simulink model "svpwm_inv_Motor_new_sent_split4"  (R2023a)
settings: Solver=daessc  StartTime=0.0  StopTime=0.62  MaxStep=2.5e-7  RelTol=1e-3
undefined symbols (not defined in the file): DiscIntNeverNeededParam
libraries: nesl_utility x37, fl_lib x34, ee_lib x21, spsMeanLib x7, simulink x6, mcbcontrolslib x4, slpidlib x4, sdl_lib x2, simulink_extras x1
(part 2 of 2)

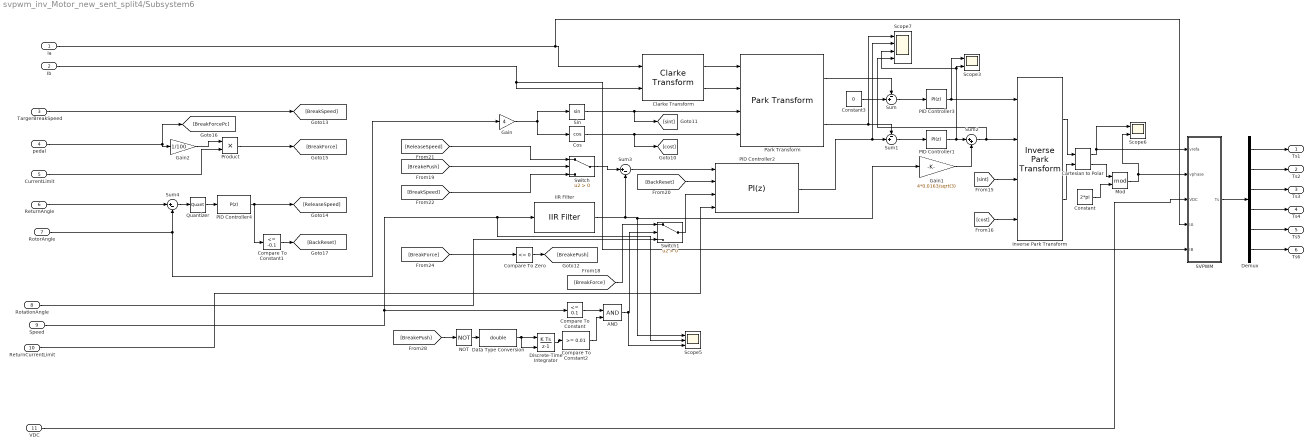
== system svpwm_inv_Motor_new_sent_split4/Subsystem6 ==
  Ia : Inport
  Ib : Inport  Port=2
  TargerBreakSpeed : Inport  Port=3
  pedal : Inport  Port=4
  CurrentLimit : Inport  Port=5
  ReturnAngle : Inport  Port=6
  RotorAngle : Inport  Port=7
  RotationAngle : Inport  Port=8
  Speed : Inport  Port=9
  ReturnCurrentLimit : Inport  Port=10
  VDC : Inport  Port=11
  AND : Logic  IconShape=distinctive  AllPortsSameDT=off  OutDataTypeStr=boolean
  Cartesian to Polar : simulink_extras/Transformations/Cartesian to Polar
  Clarke Transform : mcbcontrolslib/Clarke Transform  VariantControl=Variant2
      settings: LibrarySourceBlock=mcbhdllib/Controls/Math Transforms/Clarke Transform
  Compare To Constant : simulink/Logic and Bit Operations/Compare To Constant  relop=<=  const=0.1  OutDataTypeStr=boolean
  Compare To Constant1 : simulink/Logic and Bit Operations/Compare To Constant  relop=<=  const=-0.1  OutDataTypeStr=boolean
  Compare To Constant2 : simulink/Logic and Bit Operations/Compare To Constant  relop=>=  const=0.01  OutDataTypeStr=boolean
  Compare To Zero : simulink/Logic and Bit Operations/Compare To Zero  relop=<=  OutDataTypeStr=boolean
  Constant : Constant  Value=2*pi  SampleTime=-1
  Constant3 : Constant  Value=0  SampleTime=-1
  Cos : Trigonometry  Operator=cos
  Data Type Conversion : DataTypeConversion  OutDataTypeStr=double  SaturateOnIntegerOverflow=off  RndMeth=Floor
  Demux : Demux  Outputs=6
  Discrete-Time Integrator : DiscreteIntegrator  ExternalReset=rising  SampleTime=-1  ICPrevOutput=DiscIntNeverNeededParam  ICPrevScaledInput=DiscIntNeverNeededParam
  Gain : Gain  Gain=4
  Gain1 : Gain  Gain=4*0.0163/sqrt(3)
  Gain2 : Gain  Gain=1/100
  IIR Filter : mcbcontrolslib/IIR Filter  VariantControl=Low Pass Filter  VariantSelect=Low-pass  Filter_constant=7e-1  advancedSettings=off  Ts=50e-6  cutOff_freq=7427.2307
      settings: LibrarySourceBlock=mcbhdllib/Signal Management/IIR Filter
  Inverse Park Transform : mcbcontrolslib/Inverse Park Transform  AxisAlignment=D-axis
      settings: LibrarySourceBlock=mcbhdllib/Controls/Math Transforms/Inverse Park Transform
  Mod : Math  Operator=mod
  NOT : Logic  Operator=NOT  IconShape=distinctive  AllPortsSameDT=off  OutDataTypeStr=boolean
  PID Controller1 : slpidlib/PID Controller  Controller=PI  Form=Parallel  TimeDomain=Discrete-time  UseExternalTs=off  SampleTime=-1  IntegratorMethod=Forward Euler  FilterMethod=Forward Euler  ControllerParametersSource=internal  P=1*0.15  I=599*0.15  UseKiTs=off  D=0  N=100  UseFilter=on  TunerSelectOption=Transfer Function Based (PID Tuner App)  InitialConditionSource=internal  InitialConditionForIntegrator=0  InitialConditionForFilter=0  DifferentiatorICPrevScaledInput=0  ExternalReset=none  TrackingMode=off  Kt=1  LimitOutput=on  SatLimitsSource=internal  UpperSaturationLimit=15  LowerSaturationLimit=-15  LinearizeAsGain=off  AntiWindupMode=clamping  Kb=1  LimitIntegrator=off  UpperIntegratorSaturationLimit=inf  LowerIntegratorSaturationLimit=-inf  POutMin=[]  POutMax=[]  IOutMin=[]  IOutMax=[]  DOutMin=[]  DOutMax=[]  NOutMin=[]  NOutMax=[]  SumOutMin=[]  SumOutMax=[]  SaturationOutMin=[]  SaturationOutMax=[]  PParamMin=[]  PParamMax=[]  IParamMin=[]  IParamMax=[]  DParamMin=[]  DParamMax=[]  NParamMin=[]  NParamMax=[]  KbParamMin=[]  KbParamMax=[]  KtParamMin=[]  KtParamMax=[]  KbOutMin=[]  KbOutMax=[]  KtOutMin=[]  KtOutMax=[]  IntegratorOutMin=[]  IntegratorOutMax=[]  FilterOutMin=[]  FilterOutMax=[]  SumI1OutMin=[]  SumI1OutMax=[]  SumI2OutMin=[]  SumI2OutMax=[]  SumI3OutMin=[]  SumI3OutMax=[]  SumI4OutMin=[]  SumI4OutMax=[]  SumDOutMin=[]  SumDOutMax=[]  DifferentiatorOutMin=[]  DifferentiatorOutMax=[]  FilterDiffOutCoefMin=[]  FilterDiffOutCoefMax=[]  ReciprocalOutMin=[]  ReciprocalOutMax=[]  SumDenOutMin=[]  SumDenOutMax=[]  SumNumOutMin=[]  SumNumOutMax=[]  DivideOutMin=[]  DivideOutMax=[]  UdiffTsProdOutMin=[]  UdiffTsProdOutMax=[]  NTsProdOutMin=[]  NTsProdOutMax=[]  UintegralTsProdOutMin=[]  UintegralTsProdOutMax=[]  UngainTsProdOutMin=[]  UngainTsProdOutMax=[]  ClampingZeroOutDataTypeStr=Inherit: Inherit via back propagation  ClampingZeroOutMin=[]  ClampingZeroOutMax=[]  FilterDenConstantOutDataTypeStr=Inherit: Inherit via back propagation  FilterDenConstantOutMin=[]  FilterDenConstantOutMax=[]  PCopyOutDataTypeStr=Inherit: Inherit via back propagation  PCopyOutMin=[]  PCopyOutMax=[]  NCopyOutDataTypeStr=Inherit: Inherit via back propagation  NCopyOutMin=[]  NCopyOutMax=[]  IntegratorContinuousStateAttributes=''  IntegratorStateMustResolveToSignalObject=off  IntegratorRTWStateStorageClass=Auto  FilterContinuousStateAttributes=''  FilterStateMustResolveToSignalObject=off  FilterRTWStateStorageClass=Auto  ParallelPVariant=InternalParameters  IdealPVariant=Disabled  IVariant=InternalParameters  DVariant=Disabled  IntegratorVariant=Discrete  SatVariant=Enabled  AWVariant=DiscClampingParallel  PCopyVariant=Disabled  TRVariant=Disabled  FdbkBlocksVariant=Forward  IdealPFdbkVariant=Disabled  SatFdbkVariant=Disabled  DerivativeFilterVariant=Disabled  NVariant=Disabled  NCopyVariant=Disabled_SignalSpec  FilterICVariant=Disabled  IntegratorICVariant=InternalICs  ExternalResetVariant=Disabled  TRSumVariant=Passthrough  SumFdbkVariant=Disabled  SumVariant=Sum_PI  TsampFilterVariant=InternalTs  TsampNgainVariant=Passthrough  TsampIntegralVariant=Disabled_SignalSpec  ExternalSaturationOutDataTypeStr=Inherit: Same as second input
  PID Controller2 : slpidlib/PID Controller  Controller=PI  Form=Parallel  TimeDomain=Discrete-time  UseExternalTs=off  SampleTime=-1  IntegratorMethod=Forward Euler  FilterMethod=Forward Euler  ControllerParametersSource=internal  P=0.6  I=0  UseKiTs=off  D=0  N=100  UseFilter=on  TunerSelectOption=Transfer Function Based (PID Tuner App)  InitialConditionSource=internal  InitialConditionForIntegrator=0  InitialConditionForFilter=0  DifferentiatorICPrevScaledInput=0  ExternalReset=falling  TrackingMode=off  Kt=1  LimitOutput=on  SatLimitsSource=external  UpperSaturationLimit=45  LowerSaturationLimit=-10  LinearizeAsGain=on  AntiWindupMode=clamping  Kb=1  LimitIntegrator=off  UpperIntegratorSaturationLimit=inf  LowerIntegratorSaturationLimit=-inf  POutMin=[]  POutMax=[]  IOutMin=[]  IOutMax=[]  DOutMin=[]  DOutMax=[]  NOutMin=[]  NOutMax=[]  SumOutMin=[]  SumOutMax=[]  SaturationOutMin=[]  SaturationOutMax=[]  PParamMin=[]  PParamMax=[]  IParamMin=[]  IParamMax=[]  DParamMin=[]  DParamMax=[]  NParamMin=[]  NParamMax=[]  KbParamMin=[]  KbParamMax=[]  KtParamMin=[]  KtParamMax=[]  KbOutMin=[]  KbOutMax=[]  KtOutMin=[]  KtOutMax=[]  IntegratorOutMin=[]  IntegratorOutMax=[]  FilterOutMin=[]  FilterOutMax=[]  SumI1OutMin=[]  SumI1OutMax=[]  SumI2OutMin=[]  SumI2OutMax=[]  SumI3OutMin=[]  SumI3OutMax=[]  SumI4OutMin=[]  SumI4OutMax=[]  SumDOutMin=[]  SumDOutMax=[]  DifferentiatorOutMin=[]  DifferentiatorOutMax=[]  FilterDiffOutCoefMin=[]  FilterDiffOutCoefMax=[]  ReciprocalOutMin=[]  ReciprocalOutMax=[]  SumDenOutMin=[]  SumDenOutMax=[]  SumNumOutMin=[]  SumNumOutMax=[]  DivideOutMin=[]  DivideOutMax=[]  UdiffTsProdOutMin=[]  UdiffTsProdOutMax=[]  NTsProdOutMin=[]  NTsProdOutMax=[]  UintegralTsProdOutMin=[]  UintegralTsProdOutMax=[]  UngainTsProdOutMin=[]  UngainTsProdOutMax=[]  ClampingZeroOutDataTypeStr=Inherit: Inherit via back propagation  ClampingZeroOutMin=[]  ClampingZeroOutMax=[]  FilterDenConstantOutDataTypeStr=Inherit: Inherit via back propagation  FilterDenConstantOutMin=[]  FilterDenConstantOutMax=[]  PCopyOutDataTypeStr=Inherit: Inherit via back propagation  PCopyOutMin=[]  PCopyOutMax=[]  NCopyOutDataTypeStr=Inherit: Inherit via back propagation  NCopyOutMin=[]  NCopyOutMax=[]  IntegratorContinuousStateAttributes=''  IntegratorStateMustResolveToSignalObject=off  IntegratorRTWStateStorageClass=Auto  FilterContinuousStateAttributes=''  FilterStateMustResolveToSignalObject=off  FilterRTWStateStorageClass=Auto  ParallelPVariant=InternalParameters  IdealPVariant=Disabled  IVariant=InternalParameters  DVariant=Disabled  IntegratorVariant=Discrete  SatVariant=External  AWVariant=DiscClampingParallel  PCopyVariant=Disabled  TRVariant=Disabled  FdbkBlocksVariant=Forward  IdealPFdbkVariant=Disabled  SatFdbkVariant=Disabled  DerivativeFilterVariant=Disabled  NVariant=Disabled  NCopyVariant=Disabled_SignalSpec  FilterICVariant=Disabled  IntegratorICVariant=InternalICs  ExternalResetVariant=ExternalReset  TRSumVariant=Passthrough  SumFdbkVariant=Disabled  SumVariant=Sum_PI  TsampFilterVariant=InternalTs  TsampNgainVariant=Passthrough  TsampIntegralVariant=Disabled_SignalSpec  ExternalSaturationOutDataTypeStr=Inherit: Same as second input
  PID Controller3 : slpidlib/PID Controller  Controller=PI  Form=Parallel  TimeDomain=Discrete-time  UseExternalTs=off  SampleTime=-1  IntegratorMethod=Forward Euler  FilterMethod=Forward Euler  ControllerParametersSource=internal  P=1*0.15  I=599*0.15  UseKiTs=off  D=0  N=100  UseFilter=on  TunerSelectOption=Transfer Function Based (PID Tuner App)  InitialConditionSource=internal  InitialConditionForIntegrator=0  InitialConditionForFilter=0  DifferentiatorICPrevScaledInput=0  ExternalReset=none  TrackingMode=off  Kt=1  LimitOutput=on  SatLimitsSource=internal  UpperSaturationLimit=15  LowerSaturationLimit=-15  LinearizeAsGain=off  AntiWindupMode=clamping  Kb=1  LimitIntegrator=off  UpperIntegratorSaturationLimit=inf  LowerIntegratorSaturationLimit=-inf  POutMin=[]  POutMax=[]  IOutMin=[]  IOutMax=[]  DOutMin=[]  DOutMax=[]  NOutMin=[]  NOutMax=[]  SumOutMin=[]  SumOutMax=[]  SaturationOutMin=[]  SaturationOutMax=[]  PParamMin=[]  PParamMax=[]  IParamMin=[]  IParamMax=[]  DParamMin=[]  DParamMax=[]  NParamMin=[]  NParamMax=[]  KbParamMin=[]  KbParamMax=[]  KtParamMin=[]  KtParamMax=[]  KbOutMin=[]  KbOutMax=[]  KtOutMin=[]  KtOutMax=[]  IntegratorOutMin=[]  IntegratorOutMax=[]  FilterOutMin=[]  FilterOutMax=[]  SumI1OutMin=[]  SumI1OutMax=[]  SumI2OutMin=[]  SumI2OutMax=[]  SumI3OutMin=[]  SumI3OutMax=[]  SumI4OutMin=[]  SumI4OutMax=[]  SumDOutMin=[]  SumDOutMax=[]  DifferentiatorOutMin=[]  DifferentiatorOutMax=[]  FilterDiffOutCoefMin=[]  FilterDiffOutCoefMax=[]  ReciprocalOutMin=[]  ReciprocalOutMax=[]  SumDenOutMin=[]  SumDenOutMax=[]  SumNumOutMin=[]  SumNumOutMax=[]  DivideOutMin=[]  DivideOutMax=[]  UdiffTsProdOutMin=[]  UdiffTsProdOutMax=[]  NTsProdOutMin=[]  NTsProdOutMax=[]  UintegralTsProdOutMin=[]  UintegralTsProdOutMax=[]  UngainTsProdOutMin=[]  UngainTsProdOutMax=[]  ClampingZeroOutDataTypeStr=Inherit: Inherit via back propagation  ClampingZeroOutMin=[]  ClampingZeroOutMax=[]  FilterDenConstantOutDataTypeStr=Inherit: Inherit via back propagation  FilterDenConstantOutMin=[]  FilterDenConstantOutMax=[]  PCopyOutDataTypeStr=Inherit: Inherit via back propagation  PCopyOutMin=[]  PCopyOutMax=[]  NCopyOutDataTypeStr=Inherit: Inherit via back propagation  NCopyOutMin=[]  NCopyOutMax=[]  IntegratorContinuousStateAttributes=''  IntegratorStateMustResolveToSignalObject=off  IntegratorRTWStateStorageClass=Auto  FilterContinuousStateAttributes=''  FilterStateMustResolveToSignalObject=off  FilterRTWStateStorageClass=Auto  ParallelPVariant=InternalParameters  IdealPVariant=Disabled  IVariant=InternalParameters  DVariant=Disabled  IntegratorVariant=Discrete  SatVariant=Enabled  AWVariant=DiscClampingParallel  PCopyVariant=Disabled  TRVariant=Disabled  FdbkBlocksVariant=Forward  IdealPFdbkVariant=Disabled  SatFdbkVariant=Disabled  DerivativeFilterVariant=Disabled  NVariant=Disabled  NCopyVariant=Disabled_SignalSpec  FilterICVariant=Disabled  IntegratorICVariant=InternalICs  ExternalResetVariant=Disabled  TRSumVariant=Passthrough  SumFdbkVariant=Disabled  SumVariant=Sum_PI  TsampFilterVariant=InternalTs  TsampNgainVariant=Passthrough  TsampIntegralVariant=Disabled_SignalSpec  ExternalSaturationOutDataTypeStr=Inherit: Same as second input
  PID Controller4 : slpidlib/PID Controller  Controller=P  Form=Parallel  TimeDomain=Discrete-time  UseExternalTs=off  SampleTime=-1  IntegratorMethod=Forward Euler  FilterMethod=Forward Euler  ControllerParametersSource=internal  P=50  I=50  UseKiTs=off  D=0  N=100  UseFilter=on  TunerSelectOption=Transfer Function Based (PID Tuner App)  InitialConditionSource=internal  InitialConditionForIntegrator=0  InitialConditionForFilter=0  DifferentiatorICPrevScaledInput=0  ExternalReset=rising  TrackingMode=off  Kt=1  LimitOutput=on  SatLimitsSource=internal  UpperSaturationLimit=35  LowerSaturationLimit=-315  LinearizeAsGain=on  AntiWindupMode=clamping  Kb=1  LimitIntegrator=off  UpperIntegratorSaturationLimit=inf  LowerIntegratorSaturationLimit=-inf  POutMin=[]  POutMax=[]  IOutMin=[]  IOutMax=[]  DOutMin=[]  DOutMax=[]  NOutMin=[]  NOutMax=[]  SumOutMin=[]  SumOutMax=[]  SaturationOutMin=[]  SaturationOutMax=[]  PParamMin=[]  PParamMax=[]  IParamMin=[]  IParamMax=[]  DParamMin=[]  DParamMax=[]  NParamMin=[]  NParamMax=[]  KbParamMin=[]  KbParamMax=[]  KtParamMin=[]  KtParamMax=[]  KbOutMin=[]  KbOutMax=[]  KtOutMin=[]  KtOutMax=[]  IntegratorOutMin=[]  IntegratorOutMax=[]  FilterOutMin=[]  FilterOutMax=[]  SumI1OutMin=[]  SumI1OutMax=[]  SumI2OutMin=[]  SumI2OutMax=[]  SumI3OutMin=[]  SumI3OutMax=[]  SumI4OutMin=[]  SumI4OutMax=[]  SumDOutMin=[]  SumDOutMax=[]  DifferentiatorOutMin=[]  DifferentiatorOutMax=[]  FilterDiffOutCoefMin=[]  FilterDiffOutCoefMax=[]  ReciprocalOutMin=[]  ReciprocalOutMax=[]  SumDenOutMin=[]  SumDenOutMax=[]  SumNumOutMin=[]  SumNumOutMax=[]  DivideOutMin=[]  DivideOutMax=[]  UdiffTsProdOutMin=[]  UdiffTsProdOutMax=[]  NTsProdOutMin=[]  NTsProdOutMax=[]  UintegralTsProdOutMin=[]  UintegralTsProdOutMax=[]  UngainTsProdOutMin=[]  UngainTsProdOutMax=[]  ClampingZeroOutDataTypeStr=Inherit: Inherit via back propagation  ClampingZeroOutMin=[]  ClampingZeroOutMax=[]  FilterDenConstantOutDataTypeStr=Inherit: Inherit via back propagation  FilterDenConstantOutMin=[]  FilterDenConstantOutMax=[]  PCopyOutDataTypeStr=Inherit: Inherit via back propagation  PCopyOutMin=[]  PCopyOutMax=[]  NCopyOutDataTypeStr=Inherit: Inherit via back propagation  NCopyOutMin=[]  NCopyOutMax=[]  IntegratorContinuousStateAttributes=''  IntegratorStateMustResolveToSignalObject=off  IntegratorRTWStateStorageClass=Auto  FilterContinuousStateAttributes=''  FilterStateMustResolveToSignalObject=off  FilterRTWStateStorageClass=Auto  ParallelPVariant=InternalParameters  IdealPVariant=Disabled  IVariant=Disabled  DVariant=Disabled  IntegratorVariant=Disabled  SatVariant=Enabled  AWVariant=Disabled  PCopyVariant=Disabled  TRVariant=Disabled  FdbkBlocksVariant=Forward  IdealPFdbkVariant=Disabled  SatFdbkVariant=Disabled  DerivativeFilterVariant=Disabled  NVariant=Disabled  NCopyVariant=Disabled_SignalSpec  FilterICVariant=Disabled  IntegratorICVariant=Disabled  ExternalResetVariant=Disabled  TRSumVariant=Passthrough  SumFdbkVariant=Disabled  SumVariant=Passthrough_P  TsampFilterVariant=InternalTs  TsampNgainVariant=Passthrough  TsampIntegralVariant=Disabled_SignalSpec  ExternalSaturationOutDataTypeStr=Inherit: Same as second input
  Park Transform : mcbcontrolslib/Park Transform  AxisAlignment=D-axis
      settings: LibrarySourceBlock=mcbhdllib/Controls/Math Transforms/Park Transform
  Product : Product
  Quantizer : Quantizer  QuantizationInterval=0.1
  SVPWM : MATLAB Function  TreatAsAtomicUnit=on
  Scope3 : Scope  NumInputPorts=2
  Scope5 : Scope  NumInputPorts=3
  Scope6 : Scope  NumInputPorts=2
  Scope7 : Scope  NumInputPorts=4
  Sin : Trigonometry
  Sum : Sum  Inputs=-+|
  Sum1 : Sum  Inputs=-+|
  Sum2 : Sum  Inputs=|++
  Sum3 : Sum  Inputs=|+-
  Sum4 : Sum  Inputs=|+-
  Switch : Switch  Criteria=u2 > Threshold  SaturateOnIntegerOverflow=off  InputSameDT=off
  Switch1 : Switch  Criteria=u2 > Threshold  SaturateOnIntegerOverflow=off  InputSameDT=off
  Ts1 : Outport
  Ts2 : Outport  Port=2
  Ts3 : Outport  Port=3
  Ts4 : Outport  Port=4
  Ts5 : Outport  Port=5
  Ts6 : Outport  Port=6
  wires:
  TargerBreakSpeed/1 -> [BreakSpeed]
  RotationAngle/1 -> Switch1/3
  Switch1/1 -> PID Controller2/3
  Ia/1 -> SVPWM/4(IA), Clarke Transform/1
  Switch/1 -> Sum3/1
  Compare To Constant2/1 -> AND/2
  [BreakePush] -> Switch/2
  [sint] -> Inverse Park Transform/3
  [ReleaseSpeed] -> Switch/1
  Sum3/1 -> PID Controller2/1
  [cost] -> Inverse Park Transform/4
  Sum4/1 -> Quantizer/1
  Speed/1 -> IIR Filter/1, Scope5/2, Compare To Constant/1
  Discrete-Time Integrator/1 -> Compare To Constant2/1
  Gain/1 -> Cos/1, Sin/1
  NOT/1 -> Data Type Conversion/1
  AND/1 -> Scope5/3, Switch1/2
  Sin/1 -> Park Transform/3, [sint]
  pedal/1 -> Gain2/1, [BreakForcePc]
  ReturnCurrentLimit/1 -> PID Controller2/4
  ReturnAngle/1 -> Sum4/1
  Park Transform/2 -> Scope7/1, Sum1/1
  Compare To Constant/1 -> AND/1
  IIR Filter/1 -> Gain1/1, Scope5/1, Sum3/2
  Gain2/1 -> Product/1
  Sum1/1 -> PID Controller1/1
  Mod/1 -> Scope6/2, SVPWM/2(vphase)
  CurrentLimit/1 -> Product/2
  Product/1 -> [BreakForce]
  PID Controller3/1 -> Scope3/1, Inverse Park Transform/1
  Ib/1 -> SVPWM/5(IB), Clarke Transform/2
  [BackReset] -> PID Controller2/2
  Clarke Transform/1 -> Park Transform/1
  Cos/1 -> [cost], Park Transform/4
  RotorAngle/1 -> Gain/1, Sum4/2
  PID Controller2/1 -> Sum1/2, Scope7/2
  PID Controller1/1 -> Scope7/3, Scope3/2, Sum2/1
  Constant3/1 -> Sum/2
  [BreakForce] -> Compare To Zero/1
  Cartesian to Polar/1 -> Scope6/1, SVPWM/1(vrefa)
  Sum2/1 -> Scope7/4, Inverse Park Transform/2
  VDC/1 -> SVPWM/3(VDC)
  Inverse Park Transform/1 -> Cartesian to Polar/1
  PID Controller4/1 -> [ReleaseSpeed], Compare To Constant1/1
  Sum/1 -> PID Controller3/1
  Inverse Park Transform/2 -> Cartesian to Polar/2
  Data Type Conversion/1 -> Discrete-Time Integrator/2, Discrete-Time Integrator/1
  Cartesian to Polar/2 -> Mod/1
  Gain1/1 -> Sum2/2
  Compare To Zero/1 -> [BreakePush]
  Constant/1 -> Mod/2
  Quantizer/1 -> PID Controller4/1
  [BreakForce] -> Switch1/1
  Park Transform/1 -> Sum/1
  Compare To Constant1/1 -> [BackReset]
  [BreakePush] -> NOT/1
  Clarke Transform/2 -> Park Transform/2
  [BreakSpeed] -> Switch/3
  SVPWM/1(Ts) -> Demux/1
  Demux/1 -> Ts1/1
  Demux/2 -> Ts2/1
  Demux/3 -> Ts3/1
  Demux/4 -> Ts4/1
  Demux/5 -> Ts5/1
  Demux/6 -> Ts6/1

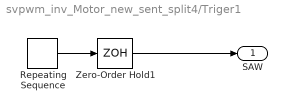
== system svpwm_inv_Motor_new_sent_split4/Triger1 ==
  Repeating Sequence : simulink/Sources/Repeating Sequence  rep_seq_t=[0 40e-6 80e-6]  rep_seq_y=[0 5000 0]
  Zero-Order Hold1 : ZeroOrderHold  SampleTime=2.5e-7
  SAW : Outport  VectorParamsAs1DForOutWhenUnconnected=off
  wires:
  Zero-Order Hold1/1 -> SAW/1
  Repeating Sequence/1 -> Zero-Order Hold1/1

== matlab function svpwm_inv_Motor_new_sent_split4/Subsystem6/SVPWM ==
  data: vrefa input; vphase input; VDC input; IA input; IB input; Ts output
%function [Ts1,Ts2,Ts3,Ts4,Ts5,Ts6] = fcn(vrefa,vphase,VDC,IA,IB)
function Ts   = fcn(vrefa,vphase,VDC,IA,IB)
%время 1/2 ШИМ периода
dt=80e-6;


%алгоритм формирования векторной ШИМ  мертвым веменем dead [мкс]
dead=0.75;
dead=dead/(dt*1e6);
a=vphase;
v2=vrefa;
if a>=0 && a<pi/3 
    n=1;
elseif  a>=pi/3 && a<2*pi/3 
    n=2;
elseif  a>=2*pi/3 && a<pi 
    n=3;
elseif  a>=pi && a<4*pi/3 
    n=4;
elseif  a>=4*pi/3 && a<5*pi/3 
    n=5;
else n=6;

end

a_cor=a-(n-1)*pi/3;

T1 = (v2/VDC)*sin(pi/3-a_cor)/sin(pi/3);
T2 = (v2/VDC)*sin(a_cor)/sin(pi/3);
T0=1-T1-T2;
Ta1=0; Ta3=0; Ta5=0; 
switch n
    case 1
        
        Ta1=T1+T2+T0/2;
        
        Ta3=T2+T0/2;
       
        Ta5=T0/2;
       
    case 2
        
        Ta1=T1+T0/2;
        
        Ta3=T1+T2+T0/2;
    
        Ta5=T0/2;       
        
    case 3
        
        Ta1=T0/2;
       
        Ta3=T1+T2+T0/2;
       
        Ta5=T2+T0/2;    
        
    case 4
        
        Ta1=T0/2;
       
        Ta3=T1+T0/2;
       
        Ta5=T1+T2+T0/2;   
       
    case 5
        
        Ta1=T2+T0/2;
        
        Ta3=T0/2;
        
        Ta5=T1+T2+T0/2;     
        
    case 6
        
        Ta1=T1+T2+T0/2;
        
        Ta3=T0/2;
     
        Ta5=T1+T0/2;    
        
end

if (Ta1 >0.95)
    Ta1 = 0.95;
elseif (Ta1 < 0.05)
        Ta1 = 0.05;
end

if (Ta3 >0.95)
    Ta3 = 0.95;
elseif (Ta3 < 0.05)
        Ta3 = 0.05;
end

if (Ta5 >0.95)
    Ta5 = 0.95;
elseif (Ta5 < 0.05)
        Ta5 = 0.05;
end


Ts1=(Ta1)-dead/2; 
Ts3=(Ta3)-dead/2; 
Ts5=(Ta5)-dead/2;
Ts2=(Ta1)+dead/2; 
Ts4=(Ta3)+dead/2; 
Ts6=(Ta5)+dead/2;


if (IA>0) 
    Ts1=Ts1+dead/2;
    Ts2=Ts2+dead/2;
else
    Ts1=Ts1-dead/2;
    Ts2=Ts2-dead/2;           
end
if (IB>0) 
    Ts3=Ts3+dead/2;
    Ts4=Ts4+dead/2;
else
    Ts3=Ts3-dead/2;
    Ts4=Ts4-dead/2; 
end  
if ((-IA-IB)>0) 
    Ts5=Ts5+dead/2;
    Ts6=Ts6+dead/2;
else
    Ts5=Ts5-dead/2;
    Ts6=Ts6-dead/2;           
end

Ts = [Ts1,Ts2,Ts3,Ts4,Ts5,Ts6];
return;
